simulink model "maglev_demo"  (Simulink 6.0)
settings: Solver=ode23  SolverMode=SingleTasking  StartTime=0.0  StopTime=5  FixedStep=1e-3  MaxStep=0.001  RelTol=1e-3  AbsTol=1e-5
PreLoadFcn:
  | load maglev_demo
undefined symbols (not defined in the file or in its folder): Kd, Ki, Kp, Ts
libraries: srolib x1
settings Model: CovMetricSettings=d  Creator=Sehnal  LastModifiedBy=rlandy  ExtModeTrigDuration=5000  ExtModeTrigLevel=0.500000  BufferReuse=off
settings DataIOCC: LimitDataPoints=off  SaveOutput=off  SaveTime=off  SignalLoggingName=sigsOut
settings OptimizationCC: BlockReduction=off  BooleanDataType=off  InlineInvariantSignals=off  OptimizeBlockIOStorage=off  BufferReuse=off  ExpressionFolding=off  FoldNonRolledExpr=off  LocalBlockOutputs=off
settings DebuggingCC: CheckExecutionContextPreStartOutputMsg=on  CheckExecutionContextRuntimeOutputMsg=on  SolverPrmCheckMsg=none
settings HardwareCC: TargetUnknown=on
settings ModelReferenceCC: UpdateModelReferenceTargets=IfOutOfDate
settings RTWCC: SystemTargetFile=rtwin.tlc  TemplateMakefile=rtwintmf  RetainRTWFile=on  ProcessScript=rtwin_make_rtw_hook
settings RTWinTargetCC: TargetFcnLib=ansi_tfl_tmw.mat  GenFloatMathFcnCalls=ANSI_C  ModelReferenceCompliant=off  MatFileLogging=on  CCOptimize=on
settings SFSimCC: SFSimApplyToAllLibs=on  SFSimBuildMode=Incremental

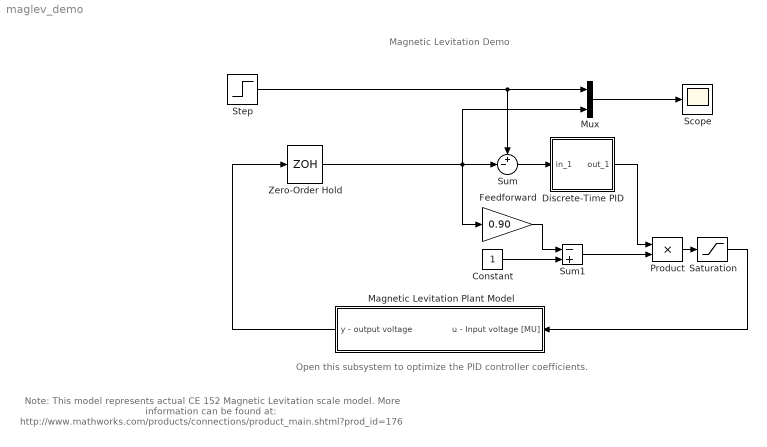
== system maglev_demo ==
  note: Note: This model represents actual CE 152 Magnetic Levitation scale model. More information can be found at:
      |           http://www.mathworks.com/products/connections/product_main.shtml?prod_id=176
  note: Magnetic Levitation Demo
  note: Open this subsystem to optimize the PID controller coefficients.
  Constant : Constant
  Discrete-Time PID : Subsystem  PropExecContextAcrossSSBoundary=on  mask(PID){Kp=Kp, Ki=Ki, Kd=Kd, Ts=Ts}
      mask prompts: Ts "Sample time:"
      mask help: Discrete-time PID controller with limited integrator
      mask Display: disp('PID');
  Feedforward : Gain  Gain=0.90  SaturateOnIntegerOverflow=on
  Magnetic Levitation Plant Model : Subsystem  Orientation=left  PropExecContextAcrossSSBoundary=on
  Mux : Mux  Inputs=2
  Product : Product  SaturateOnIntegerOverflow=on  InputSameDT=on
  Saturation : Saturate  UpperLimit=1  LowerLimit=0  ZeroCross=off
  Scope : Scope
      settings: TimeRange=5  YMin=-0.0227122  YMax=1.027  MaxDataPoints=250  SampleInput=on  SampleTime=0.02
  Step : Step  Time=0  SampleTime=0
  Sum : Sum  Inputs=+-|  SaturateOnIntegerOverflow=on  InputSameDT=on
  Sum1 : Sum  Inputs=-+  SaturateOnIntegerOverflow=on  InputSameDT=on
  Zero-Order Hold : ZeroOrderHold  SampleTime=Ts
  wires:
  Constant/1 -> Sum1/2
  Sum1/1 -> Product/2
  Feedforward/1 -> Sum1/1
  Sum/1 -> Discrete-Time PID/1(in_1)
  Discrete-Time PID/1(out_1) -> Product/1
  Zero-Order Hold/1 -> Sum/2, Feedforward/1, Mux/2
  Mux/1 -> Scope/1
  Product/1 -> Saturation/1
  Magnetic Levitation Plant Model/1(y - output voltage) -> Zero-Order Hold/1
  Saturation/1 -> Magnetic Levitation Plant Model/1(u - Input voltage [MU])
  Step/1 -> Mux/1, Sum/1

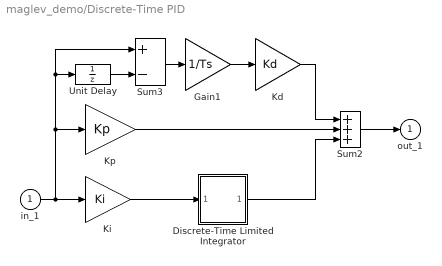
== system maglev_demo/Discrete-Time PID ==
  in_1 : Inport  LatchInput=off
  Discrete-Time Limited Integrator : Subsystem  PropExecContextAcrossSSBoundary=on  mask(Discrete-Time Limited Integrator.){@1=0, @2=2, @3=0, @4=Ts}
      mask prompts: @1 "Lower bound:"; @2 "Upper bound:"; @3 "Initial condition:"; @4 "Sampling Time:"
      mask help: Discrete-Time Limited Integrator.
      mask init:
      | lower_limit=@1;upper_limit=@2;X0=@3;Ts=@4;
      mask Help: Discrete-Time Limited Integrator. Unmask to see details.
      mask Display: plot(-1,-0.2,3.5,1.2,[0,1,2,2.9],[0,0,1,1],[0,1],[0.5,0.5], [.5,.5], [.8,.6], [.05,.35,.05,.35],[.4,.4,.2,.2], [.45,.65],[.3,.3], [.9,.9],[.2,.4]);
  Gain1 : Gain  Gain=1/Ts  SaturateOnIntegerOverflow=on
  Kd : Gain  Gain=Kd  SaturateOnIntegerOverflow=on
  Ki : Gain  Gain=Ki  SaturateOnIntegerOverflow=on
  Kp : Gain  Gain=Kp  SaturateOnIntegerOverflow=on
  Sum2 : Sum  Inputs=+++  SaturateOnIntegerOverflow=on  InputSameDT=on
  Sum3 : Sum  Inputs=+-  SaturateOnIntegerOverflow=on  InputSameDT=on
  Unit Delay : UnitDelay  SampleTime=Ts
  out_1 : Outport  InitialOutput=0
  wires:
  Unit Delay/1 -> Sum3/2
  Kd/1 -> Sum2/1
  Kp/1 -> Sum2/2
  Sum2/1 -> out_1/1
  Sum3/1 -> Gain1/1
  Gain1/1 -> Kd/1
  in_1/1 -> Ki/1, Sum3/1, Unit Delay/1, Kp/1
  Ki/1 -> Discrete-Time Limited Integrator/1(in_1)
  Discrete-Time Limited Integrator/1(out_1) -> Sum2/3

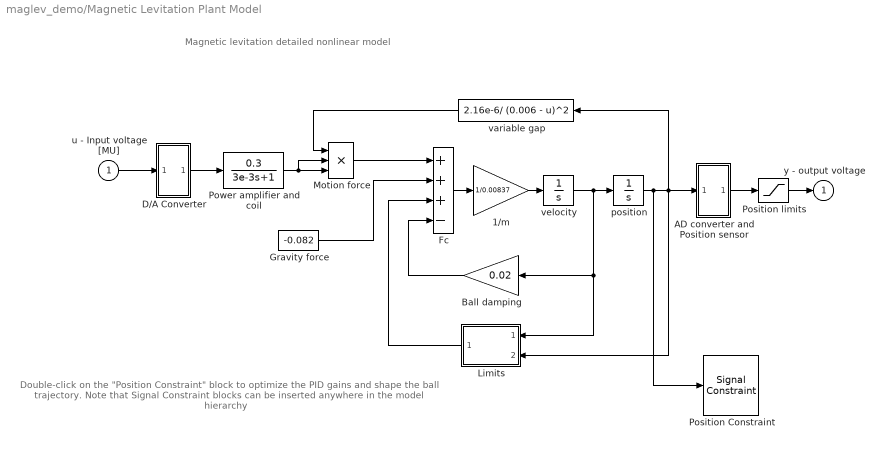
== system maglev_demo/Magnetic Levitation Plant Model ==
  note: Magnetic levitation
      | detailed nonlinear model
  note: Double-click on the "Position Constraint" block to optimize
      | the PID gains and shape the ball trajectory.
      |
      | Note that Signal Constraint blocks can be inserted
      | anywhere in the model hierarchy
  u - Input voltage [MU] : Inport  LatchInput=off
  1/m : Gain  Gain=1/0.00837  SaturateOnIntegerOverflow=on
  AD converter and Position sensor : Subsystem  PropExecContextAcrossSSBoundary=on
      mask Display: disp('A/D')
  Ball damping : Gain  Orientation=left  Gain=0.02  SaturateOnIntegerOverflow=on
  D/A Converter : Subsystem  PropExecContextAcrossSSBoundary=on
      mask Display: disp('D/A')
  Fc : Sum  Inputs=+++-  SaturateOnIntegerOverflow=on  InputSameDT=on
  Gravity force : Constant  Value=-0.082
  Limits : Subsystem  Orientation=left  PropExecContextAcrossSSBoundary=on
      mask Display: disp('LIMIT')
  Motion force : Product  Inputs=3  SaturateOnIntegerOverflow=on  InputSameDT=on
  Position limits : Saturate  UpperLimit=0.998  LowerLimit=0  ZeroCross=off
  Position Constraint : srolib/Signal Constraint  DialogPosition=[0.0109375 0.21875 0.45 0.3095703125]  SaveIn=workspace  SaveAs=maglev_optim  LogID=SRO_DataLog_1
  Power amplifier and coil : TransferFcn  Numerator=[0.3]  Denominator=[3e-3 1]
  position : Integrator  LimitOutput=on  UpperSaturationLimit=0.005  LowerSaturationLimit=0  ZeroCross=off
  variable gap : Fcn  Orientation=left  Expr=2.16e-6/ (0.006 - u)^2
  velocity : Integrator  ZeroCross=off
  y - output voltage : Outport
  wires:
  velocity/1 -> Ball damping/1, Limits/1(velocity), position/1
  Ball damping/1 -> Fc/4
  variable gap/1 -> Motion force/1
  1/m/1 -> velocity/1
  Fc/1 -> 1/m/1
  Motion force/1 -> Fc/1
  Gravity force/1 -> Fc/2
  D/A Converter/1(out_1) -> Power amplifier and coil/1
  u - Input voltage [MU]/1 -> D/A Converter/1(in_1)
  AD converter and Position sensor/1(out_1) -> Position limits/1
  position/1 -> Limits/2(position), variable gap/1, AD converter and Position sensor/1(in_1), Position Constraint/1
  Limits/1(force) -> Fc/3
  Power amplifier and coil/1 -> Motion force/3, Motion force/2
  Position limits/1 -> y - output voltage/1

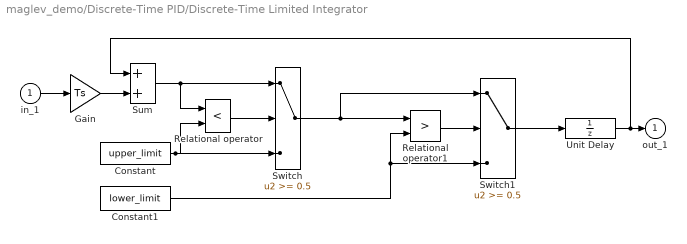
== system maglev_demo/Discrete-Time PID/Discrete-Time Limited Integrator ==
  in_1 : Inport  LatchInput=off
  Constant : Constant  Value=upper_limit
  Constant1 : Constant  Value=lower_limit
  Gain : Gain  Gain=Ts  SaturateOnIntegerOverflow=on
  Relational operator : RelationalOperator  Operator=<  InputSameDT=on
  Relational operator1 : RelationalOperator  Operator=>  InputSameDT=on
  Sum : Sum  SaturateOnIntegerOverflow=on  InputSameDT=on
  Switch : Switch  Threshold=0.5  InputSameDT=on
  Switch1 : Switch  Threshold=0.5  InputSameDT=on
  Unit Delay : UnitDelay  X0=X0  SampleTime=Ts
  out_1 : Outport  InitialOutput=0
  wires:
  Unit Delay/1 -> out_1/1, Sum/1
  Switch1/1 -> Unit Delay/1
  Constant1/1 -> Relational operator1/2, Switch1/3
  Relational operator1/1 -> Switch1/2
  Switch/1 -> Relational operator1/1, Switch1/1
  Constant/1 -> Switch/3, Relational operator/2
  Gain/1 -> Sum/2
  Sum/1 -> Switch/1, Relational operator/1
  Relational operator/1 -> Switch/2
  in_1/1 -> Gain/1

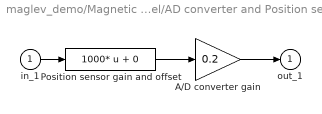
== system maglev_demo/Magnetic Levitation Plant Model/AD converter and Position sensor ==
  in_1 : Inport  LatchInput=off
  A/D converter gain : Gain  Gain=0.2  SaturateOnIntegerOverflow=on
  Position sensor gain and offset : Fcn  Expr=1000* u + 0
  out_1 : Outport
  wires:
  in_1/1 -> Position sensor gain and offset/1
  Position sensor gain and offset/1 -> A/D converter gain/1
  A/D converter gain/1 -> out_1/1

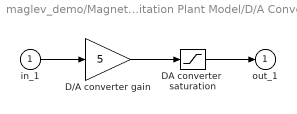
== system maglev_demo/Magnetic Levitation Plant Model/D/A Converter ==
  in_1 : Inport  LatchInput=off
  D/A converter gain : Gain  Gain=5  SaturateOnIntegerOverflow=on
  DA converter  saturation : Saturate  UpperLimit=5  LowerLimit=-5  ZeroCross=off
  out_1 : Outport
  wires:
  in_1/1 -> D/A converter gain/1
  DA converter  saturation/1 -> out_1/1
  D/A converter gain/1 -> DA converter  saturation/1

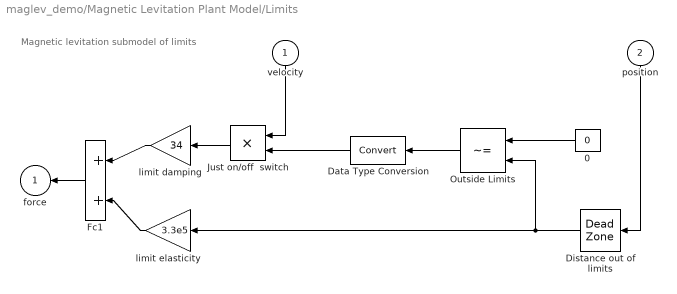
== system maglev_demo/Magnetic Levitation Plant Model/Limits ==
  note: Magnetic levitation
      | submodel of limits
  velocity : Inport  Orientation=down  LatchInput=off
  position : Inport  Orientation=down  Port=2  LatchInput=off
  0 : Constant  Orientation=left  Value=0
  Data Type Conversion : DataTypeConversion  Orientation=left  OutDataTypeMode=double  SaturateOnIntegerOverflow=on  RndMeth=Zero
  Distance out of limits : DeadZone  Orientation=left  LowerValue=0  UpperValue=0.005  ZeroCross=off  SaturateOnIntegerOverflow=on
  Fc1 : Sum  Orientation=left  SaturateOnIntegerOverflow=on  InputSameDT=on
  "Just on/off  switch " : Product  Orientation=left  SaturateOnIntegerOverflow=on  InputSameDT=on
  Outside Limits : RelationalOperator  Orientation=left  Operator=~=  InputSameDT=on
  limit damping : Gain  Orientation=left  Gain=34  SaturateOnIntegerOverflow=on
  limit elasticity : Gain  Orientation=left  Gain=3.3e5  SaturateOnIntegerOverflow=on
  force : Outport  Orientation=left
  wires:
  Distance out of limits/1 -> Outside Limits/2, limit elasticity/1
  limit damping/1 -> Fc1/1
  limit elasticity/1 -> Fc1/2
  Outside Limits/1 -> Data Type Conversion/1
  0/1 -> Outside Limits/1
  "Just on/off  switch "/1 -> limit damping/1
  velocity/1 -> "Just on/off  switch "/1
  Fc1/1 -> force/1
  position/1 -> Distance out of limits/1
  Data Type Conversion/1 -> "Just on/off  switch "/2
